simulink model "Zamora22210432HIPO"  (R2023a)
settings: Solver=ode15s  StartTime=0.0  StopTime=15  MaxStep=1e-3  RelTol=1e-3
libraries: slpidlib x1
settings Model: Creator=Asus  LastModifiedBy=Michelle
settings DataIOCC: ReturnWorkspaceOutputs=off  TimeSaveName=t
settings DebuggingCC: AlgebraicLoopMsg=none  ArtificialAlgebraicLoopMsg=none  MaxConsecutiveZCsMsg=none  ModelReferenceExtraNoncontSigs=none  OperatingPointInterfaceChecksumMismatchMsg=none

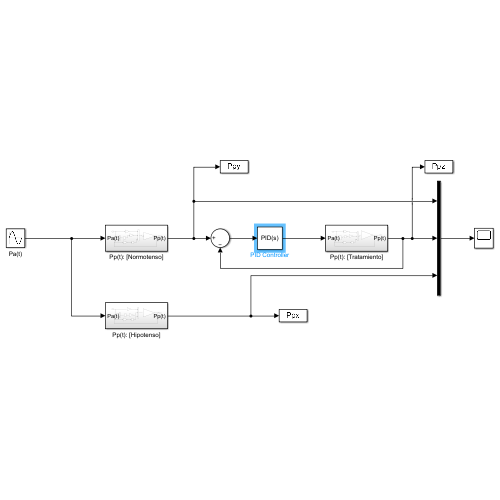
[thumbnail: Simulink's stored preview of the top-level diagram]
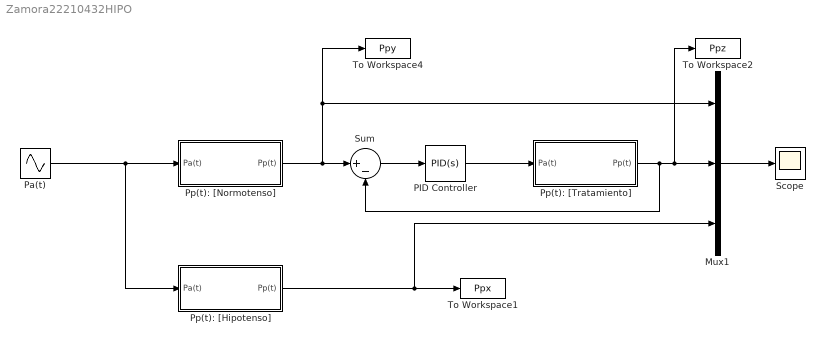
== system Zamora22210432HIPO ==
  Mux1 : Mux  Inputs=3
  PID Controller : slpidlib/PID Controller  Controller=PID  Form=Parallel  TimeDomain=Continuous-time  UseExternalTs=off  SampleTime=-1  IntegratorMethod=Forward Euler  FilterMethod=Forward Euler  ControllerParametersSource=internal  P=8.92851562535347e-05  I=1035.71406250139  UseKiTs=off  D=0  N=100  UseFilter=on  TunerSelectOption=Transfer Function Based (PID Tuner App)  InitialConditionSource=internal  InitialConditionForIntegrator=0  InitialConditionForFilter=0  DifferentiatorICPrevScaledInput=0  ExternalReset=none  TrackingMode=off  Kt=1  LimitOutput=off  SatLimitsSource=internal  UpperSaturationLimit=inf  LowerSaturationLimit=-inf  LinearizeAsGain=on  AntiWindupMode=none  Kb=1  LimitIntegrator=off  UpperIntegratorSaturationLimit=inf  LowerIntegratorSaturationLimit=-inf  POutMin=[]  POutMax=[]  IOutMin=[]  IOutMax=[]  DOutMin=[]  DOutMax=[]  NOutMin=[]  NOutMax=[]  SumOutMin=[]  SumOutMax=[]  SaturationOutMin=[]  SaturationOutMax=[]  PParamMin=[]  PParamMax=[]  IParamMin=[]  IParamMax=[]  DParamMin=[]  DParamMax=[]  NParamMin=[]  NParamMax=[]  KbParamMin=[]  KbParamMax=[]  KtParamMin=[]  KtParamMax=[]  KbOutMin=[]  KbOutMax=[]  KtOutMin=[]  KtOutMax=[]  IntegratorOutMin=[]  IntegratorOutMax=[]  FilterOutMin=[]  FilterOutMax=[]  SumI1OutMin=[]  SumI1OutMax=[]  SumI2OutMin=[]  SumI2OutMax=[]  SumI3OutMin=[]  SumI3OutMax=[]  SumI4OutMin=[]  SumI4OutMax=[]  SumDOutMin=[]  SumDOutMax=[]  DifferentiatorOutMin=[]  DifferentiatorOutMax=[]  FilterDiffOutCoefMin=[]  FilterDiffOutCoefMax=[]  ReciprocalOutMin=[]  ReciprocalOutMax=[]  SumDenOutMin=[]  SumDenOutMax=[]  SumNumOutMin=[]  SumNumOutMax=[]  DivideOutMin=[]  DivideOutMax=[]  UdiffTsProdOutMin=[]  UdiffTsProdOutMax=[]  NTsProdOutMin=[]  NTsProdOutMax=[]  UintegralTsProdOutMin=[]  UintegralTsProdOutMax=[]  UngainTsProdOutMin=[]  UngainTsProdOutMax=[]  ClampingZeroOutDataTypeStr=Inherit: Inherit via back propagation  ClampingZeroOutMin=[]  ClampingZeroOutMax=[]  FilterDenConstantOutDataTypeStr=Inherit: Inherit via back propagation  FilterDenConstantOutMin=[]  FilterDenConstantOutMax=[]  PCopyOutDataTypeStr=Inherit: Inherit via back propagation  PCopyOutMin=[]  PCopyOutMax=[]  NCopyOutDataTypeStr=Inherit: Inherit via back propagation  NCopyOutMin=[]  NCopyOutMax=[]  IntegratorContinuousStateAttributes=''  IntegratorStateMustResolveToSignalObject=off  IntegratorRTWStateStorageClass=Auto  FilterContinuousStateAttributes=''  FilterStateMustResolveToSignalObject=off  FilterRTWStateStorageClass=Auto  ParallelPVariant=InternalParameters  IdealPVariant=Disabled  IVariant=InternalParameters  DVariant=InternalParameters  IntegratorVariant=Continuous  SatVariant=Disabled  AWVariant=Passthrough  PCopyVariant=Disabled  TRVariant=Disabled  FdbkBlocksVariant=Forward  IdealPFdbkVariant=Disabled  SatFdbkVariant=Disabled  DerivativeFilterVariant=ContFilter  NVariant=InternalParameters  NCopyVariant=Disabled  FilterICVariant=InternalICsFilter  IntegratorICVariant=InternalICs  ExternalResetVariant=Disabled  TRSumVariant=Passthrough  SumFdbkVariant=Disabled  SumVariant=Sum_PID  TsampFilterVariant=InternalTs  TsampNgainVariant=Passthrough  TsampIntegralVariant=Disabled_SignalSpec  ExternalSaturationOutDataTypeStr=Inherit: Same as second input
  Pa(t) : Sin  Bias=0.8  Frequency=(2*pi)*(95/60)
  Pp(t): [Hipotenso] : Subsystem
  Pp(t): [Normotenso] : Subsystem
  Pp(t): [Tratamiento] : Subsystem
  Scope : Scope
  Sum : Sum  Inputs=|+-
  To Workspace1 : ToWorkspace  VariableName=Ppx  SampleTime=-1
  To Workspace2 : ToWorkspace  VariableName=Ppz  SampleTime=-1
  To Workspace4 : ToWorkspace  VariableName=Ppy  SampleTime=-1
  wires:
  Mux1/1 -> Scope/1
  Pa(t)/1 -> Pp(t): [Hipotenso]/1(Pa(t)), Pp(t): [Normotenso]/1(Pa(t))
  Pp(t): [Normotenso]/1(Pp(t)) -> Mux1/1, To Workspace4/1, Sum/1
  Sum/1 -> PID Controller/1
  PID Controller/1 -> Pp(t): [Tratamiento]/1(Pa(t))
  Pp(t): [Tratamiento]/1(Pp(t)) -> Mux1/2, To Workspace2/1, Sum/2
  Pp(t): [Hipotenso]/1(Pp(t)) -> Mux1/3, To Workspace1/1

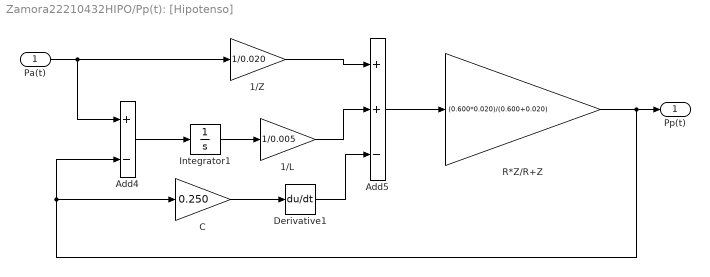
== system Zamora22210432HIPO/Pp(t): [Hipotenso] ==
  Pa(t) : Inport
  1/L : Gain  Gain=1/0.005
  1/Z : Gain  Gain=1/0.020
  Add4 : Sum  Inputs=+-
  Add5 : Sum  Inputs=++-
  C : Gain  Gain=0.250
  Derivative1 : Derivative
  Integrator1 : Integrator
  R*Z/R+Z : Gain  Gain=(0.600*0.020)/(0.600+0.020)
  Pp(t) : Outport  VectorParamsAs1DForOutWhenUnconnected=off
  wires:
  1/Z/1 -> Add5/1
  Derivative1/1 -> Add5/3
  C/1 -> Derivative1/1
  Add5/1 -> R*Z/R+Z/1
  Pa(t)/1 -> Add4/1, 1/Z/1
  R*Z/R+Z/1 -> C/1, Add4/2, Pp(t)/1
  Add4/1 -> Integrator1/1
  Integrator1/1 -> 1/L/1
  1/L/1 -> Add5/2

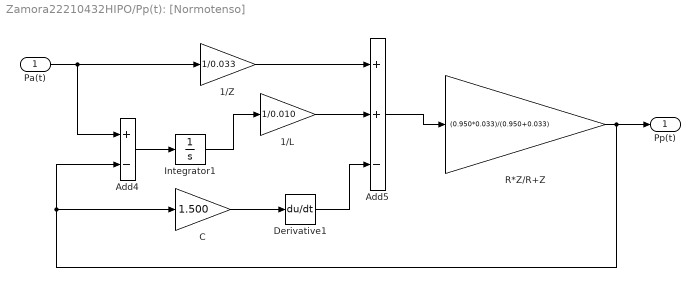
== system Zamora22210432HIPO/Pp(t): [Normotenso] ==
  Pa(t) : Inport
  1/L : Gain  Gain=1/0.010
  1/Z : Gain  Gain=1/0.033
  Add4 : Sum  Inputs=+-
  Add5 : Sum  Inputs=++-
  C : Gain  Gain=1.500
  Derivative1 : Derivative
  Integrator1 : Integrator
  R*Z/R+Z : Gain  Gain=(0.950*0.033)/(0.950+0.033)
  Pp(t) : Outport  VectorParamsAs1DForOutWhenUnconnected=off
  wires:
  1/Z/1 -> Add5/1
  Derivative1/1 -> Add5/3
  C/1 -> Derivative1/1
  Add5/1 -> R*Z/R+Z/1
  Pa(t)/1 -> Add4/1, 1/Z/1
  R*Z/R+Z/1 -> Pp(t)/1, C/1, Add4/2
  1/L/1 -> Add5/2
  Add4/1 -> Integrator1/1
  Integrator1/1 -> 1/L/1

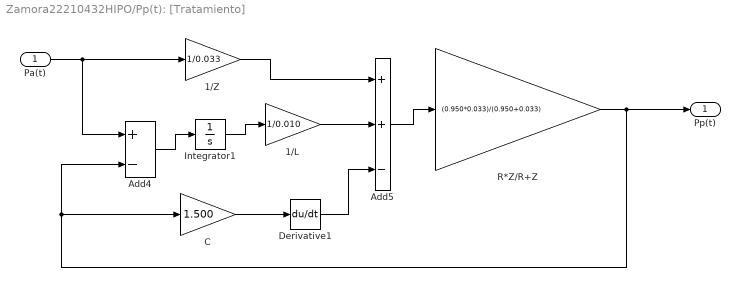
== system Zamora22210432HIPO/Pp(t): [Tratamiento] ==
  Pa(t) : Inport
  1/L : Gain  Gain=1/0.010
  1/Z : Gain  Gain=1/0.033
  Add4 : Sum  Inputs=+-
  Add5 : Sum  Inputs=++-
  C : Gain  Gain=1.500
  Derivative1 : Derivative
  Integrator1 : Integrator
  R*Z/R+Z : Gain  Gain=(0.950*0.033)/(0.950+0.033)
  Pp(t) : Outport  VectorParamsAs1DForOutWhenUnconnected=off
  wires:
  1/Z/1 -> Add5/1
  Derivative1/1 -> Add5/3
  C/1 -> Derivative1/1
  Add5/1 -> R*Z/R+Z/1
  Pa(t)/1 -> Add4/1, 1/Z/1
  R*Z/R+Z/1 -> Pp(t)/1, Add4/2, C/1
  1/L/1 -> Add5/2
  Integrator1/1 -> 1/L/1
  Add4/1 -> Integrator1/1
